simulink library "myLibrary"  (R2023b)
settings: Solver=VariableStepAuto  StartTime=0.0  StopTime=10.0  RelTol=1e-3
undefined symbols (not defined in the file): Cac_n1, ctrl1, Da, delta_slk, Discrete, dtha, ee_sli_rtmsupport, FA, gcbh, Ha, Ini, init_DCline, init_IPC, init_line, init_load, init_SG, init_shunt, init_TH, init_trafo, init_user, init_VSC, initMachineBlocks, Ka, Lf, Llkd_pu, Llkq1_pu, magnitude, NET, P, plots_step, q0, Rac_n1, Radd, Rkd_pu, Rkq1_pu, Rload_add, sim_config, sps_rtmsupport, spsSteamTurbineModel, T_DC_NET, T_global, T_IPC, T_load, T_NET, T_SG, T_shunt, T_STATCOM, T_TH, T_trafo, T_user, T_VSC, Ts, tstep, Udiff_a, V1
libraries: spsSeriesRLCBranchLib x120, eeGeneralControl x83, $bdroot x78, spsCurrentMeasurementLib x53, spsParallelRLCBranchLib x39, spsVoltageMeasurementLib x37, spsControlledVoltageSourceLib x30, simulink x29, spsFirstOrderFilterLib x18, spsMeasurementModel x13, spsThreePhaseVIMeasurementLib x5, dspsigops x4
(part 11 of 16)

== system myLibrary/GFOL/Control/Current Control ==
  Iq* : Inport
  Iq : Inport  Port=2
  Id* : Inport  Port=3
  Id : Inport  Port=4
  uq : Inport  Port=5
  ud : Inport  Port=6
  Constant : Constant  Value=T_VSC.wb
  Id1 : InportShadow  Port=4
  Integrator : Integrator  InitialCondition=initVSC.PI_idiffq
  Integrator1 : Integrator  InitialCondition=initVSC.PI_idiffd
  Iq1 : InportShadow  Port=2
  Ki : Gain  Gain=T_VSC.ki_s
  Ki1 : Gain  Gain=T_VSC.ki_s
  Kp : Gain  Gain=T_VSC.kp_s
  Kp1 : Gain  Gain=T_VSC.kp_s
  Lc : Gain  Gain=T_VSC.Lc
  Product : Product
  Product1 : Product
  Scope : Scope  NumInputPorts=2
  Sum : Sum  Inputs=|+-
  Sum1 : Sum  Inputs=|+-
  Sum2 : Sum  Inputs=+++
  Sum3 : Sum  Inputs=-++
  Sum4 : Sum
  Sum5 : Sum
  V_q_s : Outport  VectorParamsAs1DForOutWhenUnconnected=off
  V_d_s : Outport  Port=2  VectorParamsAs1DForOutWhenUnconnected=off
  wires:
  Sum2/1 -> V_q_s/1
  Sum5/1 -> Sum3/2
  Kp1/1 -> Sum5/2
  Integrator1/1 -> Sum5/1
  Ki1/1 -> Integrator1/1
  Sum1/1 -> Ki1/1, Kp1/1  "Error"
  Kp/1 -> Sum4/2
  Ki/1 -> Integrator/1
  Sum/1 -> Kp/1, Ki/1
  Lc/1 -> Product/2, Product1/1
  Id/1 -> Scope/2, Sum1/2
  Iq/1 -> Sum/2
  Iq*/1 -> Sum/1
  Constant/1 -> Lc/1
  ud/1 -> Sum3/3
  Sum4/1 -> Sum2/1
  uq/1 -> Sum2/3
  Sum3/1 -> V_d_s/1
  Product/1 -> Sum3/1
  Product1/1 -> Sum2/2
  Iq1/1 -> Product/1
  Id1/1 -> Product1/2
  Integrator/1 -> Sum4/1
  Id*/1 -> Scope/1, Sum1/1

== system myLibrary/GFOL/Control/Is ==
  Ias : Inport
  Ibs : Inport  Port=2
  Ics : Inport  Port=3
  Angle : Inport  Port=4
  Demux1 : Demux  Outputs=3
  Matriu T : Subsystem
  Mux : Mux  Inputs=3
  Product : Product  Multiplication=Matrix(*)
  Terminator : Terminator
  I_q_s : Outport  VectorParamsAs1DForOutWhenUnconnected=off
  I_d_s : Outport  Port=2  VectorParamsAs1DForOutWhenUnconnected=off
  wires:
  Product/1 -> Demux1/1
  Matriu T/1(Out1) -> Product/1
  Demux1/1 -> I_q_s/1
  Demux1/2 -> I_d_s/1
  Demux1/3 -> Terminator/1
  Angle/1 -> Matriu T/1(u)
  Mux/1 -> Product/2
  Ias/1 -> Mux/1
  Ibs/1 -> Mux/2
  Ics/1 -> Mux/3

== system myLibrary/GFOL/Control/Is1 ==
  Ias : Inport
  Ibs : Inport  Port=2
  Ics : Inport  Port=3
  Angle : Inport  Port=4
  Demux1 : Demux  Outputs=3
  Matriu T : Subsystem
  Mux : Mux  Inputs=3
  Product : Product  Multiplication=Matrix(*)
  I_q_s : Outport  VectorParamsAs1DForOutWhenUnconnected=off
  I_d_s : Outport  Port=2  VectorParamsAs1DForOutWhenUnconnected=off
  I_0_s : Outport  Port=3  VectorParamsAs1DForOutWhenUnconnected=off
  wires:
  Ics/1 -> Mux/3
  Ibs/1 -> Mux/2
  Ias/1 -> Mux/1
  Mux/1 -> Product/2
  Angle/1 -> Matriu T/1(u)
  Demux1/3 -> I_0_s/1
  Demux1/2 -> I_d_s/1
  Demux1/1 -> I_q_s/1
  Matriu T/1(Out1) -> Product/1
  Product/1 -> Demux1/1

== system myLibrary/GFOL/Control/Is3 ==
  Ias : Inport
  Ibs : Inport  Port=2
  Ics : Inport  Port=3
  Angle : Inport  Port=4
  Demux1 : Demux  Outputs=3
  Matriu T : Subsystem
  Mux : Mux  Inputs=3
  Product : Product  Multiplication=Matrix(*)
  I_q_s : Outport  VectorParamsAs1DForOutWhenUnconnected=off
  I_d_s : Outport  Port=2  VectorParamsAs1DForOutWhenUnconnected=off
  I_0_s : Outport  Port=3  VectorParamsAs1DForOutWhenUnconnected=off
  wires:
  Product/1 -> Demux1/1
  Matriu T/1(Out1) -> Product/1
  Demux1/1 -> I_q_s/1
  Demux1/2 -> I_d_s/1
  Demux1/3 -> I_0_s/1
  Angle/1 -> Matriu T/1(u)
  Mux/1 -> Product/2
  Ias/1 -> Mux/1
  Ibs/1 -> Mux/2
  Ics/1 -> Mux/3

== system myLibrary/GFOL/Control/Is4 ==
  Ias : Inport
  Ibs : Inport  Port=2
  Ics : Inport  Port=3
  Angle : Inport  Port=4
  Demux1 : Demux  Outputs=3
  Matriu T : Subsystem
  Mux : Mux  Inputs=3
  Product : Product  Multiplication=Matrix(*)
  I_q_s : Outport  VectorParamsAs1DForOutWhenUnconnected=off
  I_d_s : Outport  Port=2  VectorParamsAs1DForOutWhenUnconnected=off
  I_0_s : Outport  Port=3  VectorParamsAs1DForOutWhenUnconnected=off
  wires:
  Ics/1 -> Mux/3
  Ibs/1 -> Mux/2
  Ias/1 -> Mux/1
  Mux/1 -> Product/2
  Angle/1 -> Matriu T/1(u)
  Demux1/3 -> I_0_s/1
  Demux1/2 -> I_d_s/1
  Demux1/1 -> I_q_s/1
  Matriu T/1(Out1) -> Product/1
  Product/1 -> Demux1/1

== system myLibrary/GFOL/Control/Is5 ==
  Ias : Inport
  Ibs : Inport  Port=2
  Ics : Inport  Port=3
  Angle : Inport  Port=4
  Demux1 : Demux  Outputs=3
  Matriu T : Subsystem
  Mux : Mux  Inputs=3
  Product : Product  Multiplication=Matrix(*)
  I_q_s : Outport  VectorParamsAs1DForOutWhenUnconnected=off
  I_d_s : Outport  Port=2  VectorParamsAs1DForOutWhenUnconnected=off
  I_0_s : Outport  Port=3  VectorParamsAs1DForOutWhenUnconnected=off
  wires:
  Product/1 -> Demux1/1
  Matriu T/1(Out1) -> Product/1
  Demux1/1 -> I_q_s/1
  Demux1/2 -> I_d_s/1
  Demux1/3 -> I_0_s/1
  Angle/1 -> Matriu T/1(u)
  Mux/1 -> Product/2
  Ias/1 -> Mux/1
  Ibs/1 -> Mux/2
  Ics/1 -> Mux/3

== system myLibrary/GFOL/Control/Is7 ==
  Ias : Inport
  Ibs : Inport  Port=2
  Ics : Inport  Port=3
  Angle : Inport  Port=4
  Demux1 : Demux  Outputs=3
  Matriu T : Subsystem
  Mux : Mux  Inputs=3
  Product : Product  Multiplication=Matrix(*)
  I_q_s : Outport  VectorParamsAs1DForOutWhenUnconnected=off
  I_d_s : Outport  Port=2  VectorParamsAs1DForOutWhenUnconnected=off
  I_0_s : Outport  Port=3  VectorParamsAs1DForOutWhenUnconnected=off
  wires:
  Ics/1 -> Mux/3
  Ibs/1 -> Mux/2
  Ias/1 -> Mux/1
  Mux/1 -> Product/2
  Angle/1 -> Matriu T/1(u)
  Demux1/3 -> I_0_s/1
  Demux1/2 -> I_d_s/1
  Demux1/1 -> I_q_s/1
  Matriu T/1(Out1) -> Product/1
  Product/1 -> Demux1/1

== system myLibrary/GFOL/Control/PLL ==
  note: PLL
  U : Inport
  Ud : Inport  Port=2
  Constant : Constant  Value=0
  Constant1 : Constant
  Demux : Demux  Outputs=3
  Integrator : Integrator  InitialCondition=initVSC.thetaPLL_init
  Integrator1 : Integrator
  Ki : Gain  Gain=T_VSC.ki_pll
  Kp : Gain  Gain=T_VSC.kp_pll
  Scope1 : Scope
  Scope4 : Scope  NumInputPorts=2
  Sum : Sum  Inputs=|+-
  Sum1 : Sum  Inputs=|++
  Sum2 : Sum  Inputs=|++
  Terminator : Terminator
  Tpark : Subsystem
  wb : Gain  Gain=T_VSC.wb
  Angle : Outport
  Vzq : Outport  Port=2
  Vzd : Outport  Port=3
  w : Outport  Port=4
  wires:
  wb/1 -> Integrator/1, w/1
  Sum2/1 -> Scope1/1, wb/1
  Tpark/2(Vd) -> Vzd/1
  Constant1/1 -> Sum2/2
  Sum1/1 -> Sum2/1
  Tpark/3(0) -> Terminator/1
  Integrator/1 -> Angle/1, Tpark/4(u)
  Integrator1/1 -> Sum1/2
  Kp/1 -> Sum1/1
  Ki/1 -> Integrator1/1
  Sum/1 -> Kp/1, Ki/1
  Constant/1 -> Scope4/1, Sum/1
  Demux/1 -> Tpark/1(Va)
  Demux/3 -> Tpark/3(Vc)
  Demux/2 -> Tpark/2(Vb)
  U/1 -> Demux/1
  Tpark/1(Vq) -> Vzq/1
  Ud/1 -> Scope4/2, Sum/2

== system myLibrary/GFOL/Control/Reactive Power Control ==
  Q_ref : Inport
  id : Inport  Port=2
  iq : Inport  Port=3
  Ud : Inport  Port=4
  Uq : Inport  Port=5
  Gain : Gain  Gain=3/2
  Integrator : Integrator  InitialCondition=initVSC.idiffd
  Ki : Gain  Gain=T_VSC.ki_Q
  Kp : Gain  Gain=T_VSC.kp_Q
  Product1 : Product
  Product3 : Product
  Scope : Scope  NumInputPorts=2
  Sum : Sum  Inputs=|+-
  Sum1 : Sum  Inputs=+-
  Sum4 : Sum
  Id_ref : Outport
  wires:
  Sum4/1 -> Id_ref/1
  Sum/1 -> Kp/1, Ki/1
  Ki/1 -> Integrator/1
  Kp/1 -> Sum4/2
  Integrator/1 -> Sum4/1
  Q_ref/1 -> Scope/1, Sum/1
  Sum1/1 -> Gain/1
  Product1/1 -> Sum1/2
  Product3/1 -> Sum1/1
  Ud/1 -> Product1/1
  Uq/1 -> Product3/1
  id/1 -> Product3/2
  iq/1 -> Product1/2
  Gain/1 -> Scope/2, Sum/2

== system myLibrary/GFOL/Control/Rotació ==
  V_q_diff : Inport
  V_d_diff : Inport  Port=2
  V_0_diff : Inport  Port=3
  Angle : Inport  Port=4
  Constant{2,5..7} (4 alike) : Constant  Value=0
  Constant8 : Constant
  Demux : Demux  Outputs=3
  Display : Display
  Gain1 : Gain  Gain=-1
  Matrix Concatenate : Concatenate  NumInputs=3  Mode=Multidimensional array  ConcatenateDimension=2
  Mux{,1..3} (4 alike) : Mux  Inputs=3
  Product : Product  Multiplication=Matrix(*)
  Trigonometric Function : Trigonometry  Operator=cos
  Trigonometric Function1 : Trigonometry
  Trigonometric Function2 : Trigonometry
  Trigonometric Function3 : Trigonometry  Operator=cos
  V_alfa_diff : Outport  VectorParamsAs1DForOutWhenUnconnected=off
  V_beta_diff : Outport  Port=2  VectorParamsAs1DForOutWhenUnconnected=off
  V_0 : Outport  Port=3  VectorParamsAs1DForOutWhenUnconnected=off
  wires:
  Trigonometric Function1/1 -> Gain1/1
  Constant2/1 -> Mux1/3
  Trigonometric Function3/1 -> Mux2/2
  Constant5/1 -> Mux2/3
  Constant6/1 -> Mux3/1
  Constant7/1 -> Mux3/2
  Constant8/1 -> Mux3/3
  Mux2/1 -> Matrix Concatenate/2
  Mux3/1 -> Matrix Concatenate/3
  Mux1/1 -> Matrix Concatenate/1
  Product/1 -> Demux/1
  Demux/1 -> V_alfa_diff/1
  Demux/2 -> V_beta_diff/1
  Demux/3 -> V_0/1
  Mux/1 -> Product/2
  Matrix Concatenate/1 -> Display/1, Product/1
  V_q_diff/1 -> Mux/1
  V_d_diff/1 -> Mux/2
  V_0_diff/1 -> Mux/3
  Trigonometric Function/1 -> Mux1/1
  Gain1/1 -> Mux1/2
  Trigonometric Function2/1 -> Mux2/1
  Angle/1 -> Trigonometric Function/1, Trigonometric Function3/1, Trigonometric Function2/1, Trigonometric Function1/1

== system myLibrary/GFOL_RL/Control/Active Power Control ==
  Pac_ref : Inport
  w : Inport  Port=2
  id : Inport  Port=3
  iq : Inport  Port=4
  Ud : Inport  Port=5
  Uq : Inport  Port=6
  Constant : Constant  Value=T_VSC.wb
  Gain : Gain  Gain=3/2
  Integrator : Integrator  InitialCondition=initVSC.idiffq
  Ki : Gain  Gain=T_VSC.ki_P
  Kp : Gain  Gain=T_VSC.kp_P
  Low-Pass Filter (Discrete or Continuous)4 : eeGeneralControl/Low-Pass Filter (Discrete or Continuous)  K=1  T=T_VSC.tau_droop_f  B=inf  A=-inf  init_option=Specify as parameter  x0=T_VSC.wb  Ts=-1
  Product1 : Product
  Product3 : Product
  Scope : Scope  NumInputPorts=2
  Sum : Sum  Inputs=+-+
  Sum1 : Sum
  Sum2 : Sum  Inputs=|+-
  Sum4 : Sum
  droop : Gain  Gain=T_VSC.k_droop_f/T_VSC.wb
  Iq_ref : Outport
  wires:
  droop/1 -> Sum/3
  w/1 -> Low-Pass Filter (Discrete or Continuous)4/1
  Constant/1 -> Sum2/1
  Sum2/1 -> droop/1
  Low-Pass Filter (Discrete or Continuous)4/1 -> Sum2/2
  Uq/1 -> Product3/1
  iq/1 -> Product3/2
  Ud/1 -> Product1/1
  id/1 -> Product1/2
  Product3/1 -> Sum1/1
  Product1/1 -> Sum1/2
  Sum1/1 -> Gain/1
  Pac_ref/1 -> Scope/1, Sum/1
  Gain/1 -> Scope/2, Sum/2
  Integrator/1 -> Sum4/1
  Kp/1 -> Sum4/2
  Ki/1 -> Integrator/1
  Sum/1 -> Ki/1, Kp/1
  Sum4/1 -> Iq_ref/1

== system myLibrary/GFOL_RL/Control/Clarke Anti-Transformation ==
  V_alfa_diff : Inport
  V_beta_dfff : Inport  Port=2
  V_0_diff : Inport  Port=3
  Constant{,2,5,8} (4 alike) : Constant
  Constant1 : Constant  Value=0
  Constant3 : Constant  Value=-1/2
  Constant4 : Constant  Value=-sqrt(3)/2
  Constant6 : Constant  Value=-1/2
  Constant7 : Constant  Value=sqrt(3)/2
  Demux : Demux  Outputs=3
  Display : Display
  Math Function : Math  Operator=transpose  SignedPower=on
  Matrix Concatenate : Concatenate  NumInputs=3  Mode=Multidimensional array  ConcatenateDimension=2
  Mux{,1..3} (4 alike) : Mux  Inputs=3
  Product : Product  Multiplication=Matrix(*)
  Va_diff : Outport  VectorParamsAs1DForOutWhenUnconnected=off
  Vb_diff : Outport  Port=2  VectorParamsAs1DForOutWhenUnconnected=off
  Vc_diff : Outport  Port=3  VectorParamsAs1DForOutWhenUnconnected=off
  wires:
  Constant/1 -> Mux1/1
  Constant1/1 -> Mux1/2
  Constant2/1 -> Mux1/3
  Constant3/1 -> Mux2/1
  Constant4/1 -> Mux2/2
  Constant5/1 -> Mux2/3
  Constant6/1 -> Mux3/1
  Constant7/1 -> Mux3/2
  Constant8/1 -> Mux3/3
  Matrix Concatenate/1 -> Math Function/1
  Mux2/1 -> Matrix Concatenate/2
  Mux3/1 -> Matrix Concatenate/3
  Mux1/1 -> Matrix Concatenate/1
  Product/1 -> Demux/1
  Demux/1 -> Va_diff/1  "Va"
  Demux/2 -> Vb_diff/1  "Vb"
  Demux/3 -> Vc_diff/1  "Vc"
  Mux/1 -> Product/2
  Math Function/1 -> Display/1, Product/1
  V_alfa_diff/1 -> Mux/1  "Valfa"
  V_beta_dfff/1 -> Mux/2  "Vbeta"
  V_0_diff/1 -> Mux/3  "0"

== system myLibrary/GFOL_RL/Control/Current Control ==
  Iq* : Inport
  Iq : Inport  Port=2
  Id* : Inport  Port=3
  Id : Inport  Port=4
  uq : Inport  Port=5
  ud : Inport  Port=6
  Constant : Constant  Value=T_VSC.wb
  Id1 : InportShadow  Port=4
  Integrator : Integrator  InitialCondition=initVSC.PI_idiffq
  Integrator1 : Integrator  InitialCondition=initVSC.PI_idiffd
  Iq1 : InportShadow  Port=2
  Ki : Gain  Gain=T_VSC.ki_s
  Ki1 : Gain  Gain=T_VSC.ki_s
  Kp : Gain  Gain=T_VSC.kp_s
  Kp1 : Gain  Gain=T_VSC.kp_s
  Lc : Gain  Gain=T_VSC.Lc
  Product : Product
  Product1 : Product
  Scope : Scope  NumInputPorts=2
  Sum : Sum  Inputs=|+-
  Sum1 : Sum  Inputs=|+-
  Sum2 : Sum  Inputs=+++
  Sum3 : Sum  Inputs=-++
  Sum4 : Sum
  Sum5 : Sum
  V_q_s : Outport  VectorParamsAs1DForOutWhenUnconnected=off
  V_d_s : Outport  Port=2  VectorParamsAs1DForOutWhenUnconnected=off
  wires:
  Sum2/1 -> V_q_s/1
  Sum5/1 -> Sum3/2
  Kp1/1 -> Sum5/2
  Integrator1/1 -> Sum5/1
  Ki1/1 -> Integrator1/1
  Sum1/1 -> Ki1/1, Kp1/1  "Error"
  Kp/1 -> Sum4/2
  Ki/1 -> Integrator/1
  Sum/1 -> Kp/1, Ki/1
  Lc/1 -> Product/2, Product1/1
  Id/1 -> Scope/2, Sum1/2
  Iq/1 -> Sum/2
  Iq*/1 -> Sum/1
  Constant/1 -> Lc/1
  ud/1 -> Sum3/3
  Sum4/1 -> Sum2/1
  uq/1 -> Sum2/3
  Sum3/1 -> V_d_s/1
  Product/1 -> Sum3/1
  Product1/1 -> Sum2/2
  Iq1/1 -> Product/1
  Id1/1 -> Product1/2
  Integrator/1 -> Sum4/1
  Id*/1 -> Scope/1, Sum1/1

== system myLibrary/GFOL_RL/Control/Is ==
  Ias : Inport
  Ibs : Inport  Port=2
  Ics : Inport  Port=3
  Angle : Inport  Port=4
  Demux1 : Demux  Outputs=3
  Matriu T : Subsystem
  Mux : Mux  Inputs=3
  Product : Product  Multiplication=Matrix(*)
  Terminator : Terminator
  I_q_s : Outport  VectorParamsAs1DForOutWhenUnconnected=off
  I_d_s : Outport  Port=2  VectorParamsAs1DForOutWhenUnconnected=off
  wires:
  Product/1 -> Demux1/1
  Matriu T/1(Out1) -> Product/1
  Demux1/1 -> I_q_s/1
  Demux1/2 -> I_d_s/1
  Demux1/3 -> Terminator/1
  Angle/1 -> Matriu T/1(u)
  Mux/1 -> Product/2
  Ias/1 -> Mux/1
  Ibs/1 -> Mux/2
  Ics/1 -> Mux/3

== system myLibrary/GFOL_RL/Control/Is1 ==
  Ias : Inport
  Ibs : Inport  Port=2
  Ics : Inport  Port=3
  Angle : Inport  Port=4
  Demux1 : Demux  Outputs=3
  Matriu T : Subsystem
  Mux : Mux  Inputs=3
  Product : Product  Multiplication=Matrix(*)
  I_q_s : Outport  VectorParamsAs1DForOutWhenUnconnected=off
  I_d_s : Outport  Port=2  VectorParamsAs1DForOutWhenUnconnected=off
  I_0_s : Outport  Port=3  VectorParamsAs1DForOutWhenUnconnected=off
  wires:
  Ics/1 -> Mux/3
  Ibs/1 -> Mux/2
  Ias/1 -> Mux/1
  Mux/1 -> Product/2
  Angle/1 -> Matriu T/1(u)
  Demux1/3 -> I_0_s/1
  Demux1/2 -> I_d_s/1
  Demux1/1 -> I_q_s/1
  Matriu T/1(Out1) -> Product/1
  Product/1 -> Demux1/1

== system myLibrary/GFOL_RL/Control/Is3 ==
  Ias : Inport
  Ibs : Inport  Port=2
  Ics : Inport  Port=3
  Angle : Inport  Port=4
  Demux1 : Demux  Outputs=3
  Matriu T : Subsystem
  Mux : Mux  Inputs=3
  Product : Product  Multiplication=Matrix(*)
  I_q_s : Outport  VectorParamsAs1DForOutWhenUnconnected=off
  I_d_s : Outport  Port=2  VectorParamsAs1DForOutWhenUnconnected=off
  I_0_s : Outport  Port=3  VectorParamsAs1DForOutWhenUnconnected=off
  wires:
  Product/1 -> Demux1/1
  Matriu T/1(Out1) -> Product/1
  Demux1/1 -> I_q_s/1
  Demux1/2 -> I_d_s/1
  Demux1/3 -> I_0_s/1
  Angle/1 -> Matriu T/1(u)
  Mux/1 -> Product/2
  Ias/1 -> Mux/1
  Ibs/1 -> Mux/2
  Ics/1 -> Mux/3

== system myLibrary/GFOL_RL/Control/Is4 ==
  Ias : Inport
  Ibs : Inport  Port=2
  Ics : Inport  Port=3
  Angle : Inport  Port=4
  Demux1 : Demux  Outputs=3
  Matriu T : Subsystem
  Mux : Mux  Inputs=3
  Product : Product  Multiplication=Matrix(*)
  I_q_s : Outport  VectorParamsAs1DForOutWhenUnconnected=off
  I_d_s : Outport  Port=2  VectorParamsAs1DForOutWhenUnconnected=off
  I_0_s : Outport  Port=3  VectorParamsAs1DForOutWhenUnconnected=off
  wires:
  Ics/1 -> Mux/3
  Ibs/1 -> Mux/2
  Ias/1 -> Mux/1
  Mux/1 -> Product/2
  Angle/1 -> Matriu T/1(u)
  Demux1/3 -> I_0_s/1
  Demux1/2 -> I_d_s/1
  Demux1/1 -> I_q_s/1
  Matriu T/1(Out1) -> Product/1
  Product/1 -> Demux1/1

== system myLibrary/GFOL_RL/Control/Is5 ==
  Ias : Inport
  Ibs : Inport  Port=2
  Ics : Inport  Port=3
  Angle : Inport  Port=4
  Demux1 : Demux  Outputs=3
  Matriu T : Subsystem
  Mux : Mux  Inputs=3
  Product : Product  Multiplication=Matrix(*)
  I_q_s : Outport  VectorParamsAs1DForOutWhenUnconnected=off
  I_d_s : Outport  Port=2  VectorParamsAs1DForOutWhenUnconnected=off
  I_0_s : Outport  Port=3  VectorParamsAs1DForOutWhenUnconnected=off
  wires:
  Product/1 -> Demux1/1
  Matriu T/1(Out1) -> Product/1
  Demux1/1 -> I_q_s/1
  Demux1/2 -> I_d_s/1
  Demux1/3 -> I_0_s/1
  Angle/1 -> Matriu T/1(u)
  Mux/1 -> Product/2
  Ias/1 -> Mux/1
  Ibs/1 -> Mux/2
  Ics/1 -> Mux/3

== system myLibrary/GFOL_RL/Control/PLL ==
  note: PLL
  U : Inport
  Constant : Constant  Value=0
  Constant1 : Constant
  Demux : Demux  Outputs=3
  Integrator : Integrator  InitialCondition=initVSC.thetaPLL_init
  Integrator1 : Integrator
  Ki : Gain  Gain=T_VSC.ki_pll
  Kp : Gain  Gain=T_VSC.kp_pll
  Scope1 : Scope
  Scope4 : Scope  NumInputPorts=2
  Sum : Sum  Inputs=|+-
  Sum1 : Sum  Inputs=|++
  Sum2 : Sum  Inputs=|++
  Terminator : Terminator
  Tpark : Subsystem
  wb : Gain  Gain=T_VSC.wb
  Angle : Outport
  Vzq : Outport  Port=2
  Vzd : Outport  Port=3
  w : Outport  Port=4
  wires:
  wb/1 -> Integrator/1, w/1
  Sum2/1 -> Scope1/1, wb/1
  Tpark/2(Vd) -> Scope4/2, Sum/2, Vzd/1
  Constant1/1 -> Sum2/2
  Sum1/1 -> Sum2/1
  Tpark/3(0) -> Terminator/1
  Integrator/1 -> Angle/1, Tpark/4(u)
  Integrator1/1 -> Sum1/2
  Kp/1 -> Sum1/1
  Ki/1 -> Integrator1/1
  Sum/1 -> Kp/1, Ki/1
  Constant/1 -> Scope4/1, Sum/1
  Demux/1 -> Tpark/1(Va)
  Demux/3 -> Tpark/3(Vc)
  Demux/2 -> Tpark/2(Vb)
  U/1 -> Demux/1
  Tpark/1(Vq) -> Vzq/1

== system myLibrary/GFOL_RL/Control/Reactive Power Control ==
  Q_ref : Inport
  id : Inport  Port=2
  iq : Inport  Port=3
  Ud : Inport  Port=4
  Uq : Inport  Port=5
  Gain : Gain  Gain=3/2
  Integrator : Integrator  InitialCondition=initVSC.idiffd
  Ki : Gain  Gain=T_VSC.ki_Q
  Kp : Gain  Gain=T_VSC.kp_Q
  Product1 : Product
  Product3 : Product
  Scope : Scope  NumInputPorts=2
  Sum : Sum  Inputs=|+-
  Sum1 : Sum  Inputs=+-
  Sum4 : Sum
  Id_ref : Outport
  wires:
  Sum4/1 -> Id_ref/1
  Sum/1 -> Kp/1, Ki/1
  Ki/1 -> Integrator/1
  Kp/1 -> Sum4/2
  Integrator/1 -> Sum4/1
  Q_ref/1 -> Scope/1, Sum/1
  Sum1/1 -> Gain/1
  Product1/1 -> Sum1/2
  Product3/1 -> Sum1/1
  Ud/1 -> Product1/1
  Uq/1 -> Product3/1
  id/1 -> Product3/2
  iq/1 -> Product1/2
  Gain/1 -> Scope/2, Sum/2

== system myLibrary/GFOL_RL/Control/Rotació ==
  V_q_diff : Inport
  V_d_diff : Inport  Port=2
  V_0_diff : Inport  Port=3
  Angle : Inport  Port=4
  Constant{2,5..7} (4 alike) : Constant  Value=0
  Constant8 : Constant
  Demux : Demux  Outputs=3
  Display : Display
  Gain1 : Gain  Gain=-1
  Matrix Concatenate : Concatenate  NumInputs=3  Mode=Multidimensional array  ConcatenateDimension=2
  Mux{,1..3} (4 alike) : Mux  Inputs=3
  Product : Product  Multiplication=Matrix(*)
  Trigonometric Function : Trigonometry  Operator=cos
  Trigonometric Function1 : Trigonometry
  Trigonometric Function2 : Trigonometry
  Trigonometric Function3 : Trigonometry  Operator=cos
  V_alfa_diff : Outport  VectorParamsAs1DForOutWhenUnconnected=off
  V_beta_diff : Outport  Port=2  VectorParamsAs1DForOutWhenUnconnected=off
  V_0 : Outport  Port=3  VectorParamsAs1DForOutWhenUnconnected=off
  wires:
  Trigonometric Function1/1 -> Gain1/1
  Constant2/1 -> Mux1/3
  Trigonometric Function3/1 -> Mux2/2
  Constant5/1 -> Mux2/3
  Constant6/1 -> Mux3/1
  Constant7/1 -> Mux3/2
  Constant8/1 -> Mux3/3
  Mux2/1 -> Matrix Concatenate/2
  Mux3/1 -> Matrix Concatenate/3
  Mux1/1 -> Matrix Concatenate/1
  Product/1 -> Demux/1
  Demux/1 -> V_alfa_diff/1
  Demux/2 -> V_beta_diff/1
  Demux/3 -> V_0/1
  Mux/1 -> Product/2
  Matrix Concatenate/1 -> Display/1, Product/1
  V_q_diff/1 -> Mux/1
  V_d_diff/1 -> Mux/2
  V_0_diff/1 -> Mux/3
  Trigonometric Function/1 -> Mux1/1
  Gain1/1 -> Mux1/2
  Trigonometric Function2/1 -> Mux2/1
  Angle/1 -> Trigonometric Function/1, Trigonometric Function3/1, Trigonometric Function2/1, Trigonometric Function1/1

== system myLibrary/GFOR/Control/Clarke Anti-Transformation ==
  V_alfa_diff : Inport
  V_beta_dfff : Inport  Port=2
  V_0_diff : Inport  Port=3
  Constant{,2,5,8} (4 alike) : Constant
  Constant1 : Constant  Value=0
  Constant3 : Constant  Value=-1/2
  Constant4 : Constant  Value=-sqrt(3)/2
  Constant6 : Constant  Value=-1/2
  Constant7 : Constant  Value=sqrt(3)/2
  Demux : Demux  Outputs=3
  Display : Display
  Math Function : Math  Operator=transpose  SignedPower=on
  Matrix Concatenate : Concatenate  NumInputs=3  Mode=Multidimensional array  ConcatenateDimension=2
  Mux{,1..3} (4 alike) : Mux  Inputs=3
  Product : Product  Multiplication=Matrix(*)
  Va_diff : Outport  VectorParamsAs1DForOutWhenUnconnected=off
  Vb_diff : Outport  Port=2  VectorParamsAs1DForOutWhenUnconnected=off
  Vc_diff : Outport  Port=3  VectorParamsAs1DForOutWhenUnconnected=off
  wires:
  V_0_diff/1 -> Mux/3  "0"
  V_beta_dfff/1 -> Mux/2  "Vbeta"
  V_alfa_diff/1 -> Mux/1  "Valfa"
  Math Function/1 -> Product/1, Display/1
  Mux/1 -> Product/2
  Demux/3 -> Vc_diff/1  "Vc"
  Demux/2 -> Vb_diff/1  "Vb"
  Demux/1 -> Va_diff/1  "Va"
  Product/1 -> Demux/1
  Mux1/1 -> Matrix Concatenate/1
  Mux3/1 -> Matrix Concatenate/3
  Mux2/1 -> Matrix Concatenate/2
  Matrix Concatenate/1 -> Math Function/1
  Constant8/1 -> Mux3/3
  Constant7/1 -> Mux3/2
  Constant6/1 -> Mux3/1
  Constant5/1 -> Mux2/3
  Constant4/1 -> Mux2/2
  Constant3/1 -> Mux2/1
  Constant2/1 -> Mux1/3
  Constant1/1 -> Mux1/2
  Constant/1 -> Mux1/1

== system myLibrary/GFOR/Control/Current Control ==
  Iq* : Inport
  Iq : Inport  Port=2
  Id* : Inport  Port=3
  Id : Inport  Port=4
  uq : Inport  Port=5
  ud : Inport  Port=6
  Constant : Constant  Value=T_VSC.wb
  Id1 : InportShadow  Port=4
  Integrator : Integrator  InitialCondition=initVSC.PI_idiffq
  Integrator1 : Integrator  InitialCondition=initVSC.PI_idiffd
  Iq1 : InportShadow  Port=2
  Ki : Gain  Gain=T_VSC.ki_s
  Ki1 : Gain  Gain=T_VSC.ki_s
  Kp : Gain  Gain=T_VSC.kp_s
  Kp1 : Gain  Gain=T_VSC.kp_s
  Lc : Gain  Gain=T_VSC.Lc
  Product : Product
  Product1 : Product
  Sum : Sum  Inputs=|+-
  Sum1 : Sum  Inputs=|+-
  Sum2 : Sum  Inputs=+++
  Sum3 : Sum  Inputs=-++
  Sum4 : Sum
  Sum5 : Sum
  V_q_s : Outport  VectorParamsAs1DForOutWhenUnconnected=off
  V_d_s : Outport  Port=2  VectorParamsAs1DForOutWhenUnconnected=off
  wires:
  Id*/1 -> Sum1/1
  Integrator/1 -> Sum4/1
  Id1/1 -> Product1/2
  Iq1/1 -> Product/1
  Product1/1 -> Sum2/2
  Product/1 -> Sum3/1
  Sum3/1 -> V_d_s/1
  uq/1 -> Sum2/3
  Sum4/1 -> Sum2/1
  ud/1 -> Sum3/3
  Constant/1 -> Lc/1
  Iq*/1 -> Sum/1
  Iq/1 -> Sum/2
  Id/1 -> Sum1/2
  Lc/1 -> Product1/1, Product/2
  Sum/1 -> Ki/1, Kp/1
  Ki/1 -> Integrator/1
  Kp/1 -> Sum4/2
  Sum1/1 -> Kp1/1, Ki1/1  "Error"
  Ki1/1 -> Integrator1/1
  Integrator1/1 -> Sum5/1
  Kp1/1 -> Sum5/2
  Sum5/1 -> Sum3/2
  Sum2/1 -> V_q_s/1

== system myLibrary/GFOR/Control/Is ==
  Ias : Inport
  Ibs : Inport  Port=2
  Ics : Inport  Port=3
  Angle : Inport  Port=4
  Demux1 : Demux  Outputs=3
  Matriu T : Subsystem
  Mux : Mux  Inputs=3
  Product : Product  Multiplication=Matrix(*)
  Terminator : Terminator
  I_q_s : Outport  VectorParamsAs1DForOutWhenUnconnected=off
  I_d_s : Outport  Port=2  VectorParamsAs1DForOutWhenUnconnected=off
  wires:
  Ics/1 -> Mux/3
  Ibs/1 -> Mux/2
  Ias/1 -> Mux/1
  Mux/1 -> Product/2
  Angle/1 -> Matriu T/1(u)
  Demux1/3 -> Terminator/1
  Demux1/2 -> I_d_s/1
  Demux1/1 -> I_q_s/1
  Matriu T/1(Out1) -> Product/1
  Product/1 -> Demux1/1

== system myLibrary/GFOR/Control/Is2 ==
  Ias : Inport
  Ibs : Inport  Port=2
  Ics : Inport  Port=3
  Angle : Inport  Port=4
  Demux1 : Demux  Outputs=3
  Matriu T : Subsystem
  Mux : Mux  Inputs=3
  Product : Product  Multiplication=Matrix(*)
  I_q_s : Outport  VectorParamsAs1DForOutWhenUnconnected=off
  I_d_s : Outport  Port=2  VectorParamsAs1DForOutWhenUnconnected=off
  I_0_s : Outport  Port=3  VectorParamsAs1DForOutWhenUnconnected=off
  wires:
  Ics/1 -> Mux/3
  Ibs/1 -> Mux/2
  Ias/1 -> Mux/1
  Mux/1 -> Product/2
  Angle/1 -> Matriu T/1(u)
  Demux1/3 -> I_0_s/1
  Demux1/2 -> I_d_s/1
  Demux1/1 -> I_q_s/1
  Matriu T/1(Out1) -> Product/1
  Product/1 -> Demux1/1

== system myLibrary/GFOR/Control/PLL ==
  note: PLL
  Pref : Inport
  iq : Inport  Port=2
  uq : Inport  Port=3
  id : Inport  Port=4
  ud : Inport  Port=5
  Constant4 : Constant
  Gain5 : Gain  Gain=3/2
  Integrator2 : Integrator  InitialCondition=initVSC.thetaPLL_init
  Low-Pass Filter (Discrete or Continuous)2 : eeGeneralControl/Low-Pass Filter (Discrete or Continuous)  K=1  T=T_VSC.tau_droop_f  B=inf  A=-inf  init_option=Specify as parameter  x0=initVSC.Pref  Ts=0
  Product3 : Product
  Product5 : Product
  Scope4 : Scope  NumInputPorts=2
  Sum18 : Sum  Inputs=++|
  Sum3 : Sum
  Sum35 : Sum  Inputs=|+-
  kdroop : Gain  Gain=T_VSC.k_droop_f
  wb : Gain  Gain=T_VSC.wb
  Angle : Outport
  tag scope: w_GFOR1=global
  wires:
  Product5/1 -> Sum3/2
  Low-Pass Filter (Discrete or Continuous)2/1 -> Scope4/1, Sum35/2
  Product3/1 -> Sum3/1
  Sum35/1 -> kdroop/1
  Sum18/1 -> wb/1
  Integrator2/1 -> Angle/1
  Sum3/1 -> Gain5/1  "V_0_s"
  Constant4/1 -> Sum18/1  "w0_pu"
  kdroop/1 -> Sum18/2
  Gain5/1 -> Low-Pass Filter (Discrete or Continuous)2/1
  iq/1 -> Product3/1
  uq/1 -> Product3/2
  id/1 -> Product5/1
  ud/1 -> Product5/2
  Pref/1 -> Sum35/1, Scope4/2
  wb/1 -> [w_GFOR1], Integrator2/1

== system myLibrary/GFOR/Control/Rotació ==
  V_q_diff : Inport
  V_d_diff : Inport  Port=2
  V_0_diff : Inport  Port=3
  Angle : Inport  Port=4
  Constant{2,5..7} (4 alike) : Constant  Value=0
  Constant8 : Constant
  Demux : Demux  Outputs=3
  Display : Display
  Gain1 : Gain  Gain=-1
  Matrix Concatenate : Concatenate  NumInputs=3  Mode=Multidimensional array  ConcatenateDimension=2
  Mux{,1..3} (4 alike) : Mux  Inputs=3
  Product : Product  Multiplication=Matrix(*)
  Trigonometric Function : Trigonometry  Operator=cos
  Trigonometric Function1 : Trigonometry
  Trigonometric Function2 : Trigonometry
  Trigonometric Function3 : Trigonometry  Operator=cos
  V_alfa_diff : Outport  VectorParamsAs1DForOutWhenUnconnected=off
  V_beta_diff : Outport  Port=2  VectorParamsAs1DForOutWhenUnconnected=off
  V_0 : Outport  Port=3  VectorParamsAs1DForOutWhenUnconnected=off
  wires:
  Angle/1 -> Trigonometric Function1/1, Trigonometric Function2/1, Trigonometric Function3/1, Trigonometric Function/1
  Trigonometric Function2/1 -> Mux2/1
  Gain1/1 -> Mux1/2
  Trigonometric Function/1 -> Mux1/1
  V_0_diff/1 -> Mux/3
  V_d_diff/1 -> Mux/2
  V_q_diff/1 -> Mux/1
  Matrix Concatenate/1 -> Product/1, Display/1
  Mux/1 -> Product/2
  Demux/3 -> V_0/1
  Demux/2 -> V_beta_diff/1
  Demux/1 -> V_alfa_diff/1
  Product/1 -> Demux/1
  Mux1/1 -> Matrix Concatenate/1
  Mux3/1 -> Matrix Concatenate/3
  Mux2/1 -> Matrix Concatenate/2
  Constant8/1 -> Mux3/3
  Constant7/1 -> Mux3/2
  Constant6/1 -> Mux3/1
  Constant5/1 -> Mux2/3
  Trigonometric Function3/1 -> Mux2/2
  Constant2/1 -> Mux1/3
  Trigonometric Function1/1 -> Gain1/1

== system myLibrary/GFOR/Control/Voltage control ==
  vq_ref : Inport
  vd_ref : Inport  Port=2
  vq : Inport  Port=3
  vd : Inport  Port=4
  igq : Inport  Port=5
  igd : Inport  Port=6
  Cac : Gain  Gain=T_VSC.Cac
  Constant : Constant  Value=T_VSC.wb
  Feed-Forward filter igq : eeGeneralControl/Low-Pass Filter (Discrete or Continuous)  K=1  T=T_VSC.tau_ig  B=inf  A=-inf  init_option=Specify as parameter  x0=initVSC.igq  Ts=0
  Feed-Forward filter igq1 : eeGeneralControl/Low-Pass Filter (Discrete or Continuous)  K=1  T=T_VSC.tau_ig  B=inf  A=-inf  init_option=Specify as parameter  x0=initVSC.igd  Ts=0
  Integrator1 : Integrator  InitialCondition=initVSC.PI_vacq
  Integrator2 : Integrator  InitialCondition=initVSC.PI_vacd
  Product3 : Product  RndMeth=Zero
  Product4 : Product  RndMeth=Zero
  Scope : Scope  NumInputPorts=2
  Sum1 : Sum  Inputs=|+-
  Sum10 : Sum  Inputs=|++
  Sum2 : Sum  Inputs=+++
  Sum3 : Sum  Inputs=-+|
  Sum5 : Sum  Inputs=-++
  Sum8 : Sum  Inputs=|++
  ki : Gain  Gain=T_VSC.ki_vac
  ki2 : Gain  Gain=T_VSC.ki_vac
  kp : Gain  Gain=T_VSC.kp_vac
  kp2 : Gain  Gain=T_VSC.kp_vac
  vd1 : InportShadow  Port=4
  vq1 : InportShadow  Port=3
  iqref : Outport  VectorParamsAs1DForOutWhenUnconnected=off
  idref : Outport  Port=2  VectorParamsAs1DForOutWhenUnconnected=off
  wires:
  vd1/1 -> Product4/2
  vq1/1 -> Product3/1
  Sum8/1 -> Sum2/2
  vd/1 -> Sum3/1
  vq/1 -> Sum1/2
  ki2/1 -> Integrator2/1
  kp2/1 -> Sum10/1
  ki/1 -> Integrator1/1
  vd_ref/1 -> Sum3/2
  Sum5/1 -> idref/1
  vq_ref/1 -> Sum1/1
  Integrator1/1 -> Scope/1, Sum8/2
  Sum10/1 -> Sum5/2
  kp/1 -> Sum8/1
  Integrator2/1 -> Sum10/2, Scope/2
  Sum2/1 -> iqref/1
  Constant/1 -> Cac/1
  Cac/1 -> Product4/1, Product3/2
  Sum1/1 -> ki/1, kp/1
  Sum3/1 -> ki2/1, kp2/1
  Product3/1 -> Sum5/1
  Product4/1 -> Sum2/3
  Feed-Forward filter igq/1 -> Sum2/1
  Feed-Forward filter igq1/1 -> Sum5/3
  igd/1 -> Feed-Forward filter igq1/1
  igq/1 -> Feed-Forward filter igq/1

== system myLibrary/SG/Exciter/Exciter AC4A ==
  vref : Inport
  Vt : Inport  Port=2
  Vs : Inport  Port=3
  IC1 : InitialCondition  Value=0
  Lag-lead network Transient gain reduction : TransferFcn  Numerator=[T_SG.exc.TC 1]  Denominator=[T_SG.exc.TB 1]
  Sum2 : Sum  Inputs=+-+
  Transfer Fcn3 : TransferFcn  Numerator=[T_SG.exc.KA]  Denominator=[T_SG.exc.TA 1]
  Voltage transducer : spsFirstOrderFilterLib/First-Order Filter  FilterType=Lowpass  Tc=T_SG.exc.TR  Ts=sim_config.Ts  Initialize=on  Vac_Init=[0, 0, T_SG.fb]  Vdc_Init=initSG.Vref  PlotResponse=off  FreqRange="[0,  200,  1]"
  Vfn_pu : Outport
  wires:
  Vs/1 -> Sum2/3  "V"
  Voltage transducer/1 -> Sum2/2  "Vc"
  Vt/1 -> Voltage transducer/1  "V"
  Sum2/1 -> IC1/1  "VI"
  Lag-lead network Transient gain reduction/1 -> Transfer Fcn3/1  "VR"
  vref/1 -> Sum2/1
  Transfer Fcn3/1 -> Vfn_pu/1  "Vfn_pu"
  IC1/1 -> Lag-lead network Transient gain reduction/1

== system myLibrary/SG/Exciter/Exciter AC8C ==
  vref : Inport
  Vs : Inport  Port=2
  Vt : Inport  Port=3
  Ifd_pu : Inport  Port=4
  AC ROTATING MACHINE : Subsystem
  Divide : Product  Inputs=*/
  Gain : Gain  Gain=T_SG.exc.KP
  Gain1 : Gain  Gain=-0.577*T_SG.exc.KC  OutDataTypeStr=double
  Lag-lead network Transient gain reduction2 : TransferFcn  Numerator=[(T_SG.exc.KPR*T_SG.exc.TDR+T_SG.exc.KDR) (T_SG.exc.KPR+T_SG.exc.KIR*T_SG.exc.TDR) (T_SG.exc.KIR)]  Denominator=[T_SG.exc.TDR 1 0]
  Product : Product  OutDataTypeStr=Inherit: Same as first input
  Product1 : Product
  Sum : Sum  Inputs=+-+  InputSameDT=on  SaturateOnIntegerOverflow=on  OutDataTypeStr=Inherit: Same as first input
  Transfer Fcn3 : TransferFcn  Numerator=[T_SG.exc.KA]  Denominator=[T_SG.exc.TA 1]
  Voltage transducer : spsFirstOrderFilterLib/First-Order Filter  FilterType=Lowpass  Tc=T_SG.exc.TR  Ts=sim_config.Ts  Initialize=on  Vac_Init=[0, 0, T_SG.fb]  Vdc_Init=initSG.Vref  PlotResponse=off  FreqRange="[0,  200,  1]"
  Vt1 : InportShadow  Port=3
  Vfn_pu : Outport
  wires:
  Product1/1 -> Product/2  "V_B"
  Sum/1 -> Lag-lead network Transient gain reduction2/1  "VR"
  Vt/1 -> Voltage transducer/1  "V"
  Vt1/1 -> Gain/1  "V"
  Vs/1 -> Sum/3
  Gain/1 -> Divide/2, Product1/2  "V_E"
  Gain1/1 -> Product1/1  "F_EX"
  vref/1 -> Sum/1
  Voltage transducer/1 -> Sum/2  "Vc"
  Lag-lead network Transient gain reduction2/1 -> Transfer Fcn3/1  "V_M"
  Product/1 -> AC ROTATING MACHINE/1(EFE)
  Ifd_pu/1 -> AC ROTATING MACHINE/2(IFD)
  AC ROTATING MACHINE/2(VFE) -> Divide/1
  AC ROTATING MACHINE/1(EFD) -> Vfn_pu/1
  Divide/1 -> Gain1/1  "F_EX"
  Transfer Fcn3/1 -> Product/1  "V_A"

== system myLibrary/SG/Exciter/Exciter ST1 ==
  vref : Inport
  Vt : Inport  Port=2
  Vs : Inport  Port=3
  IC1 : InitialCondition  Value=0
  Lag-lead network Transient gain reduction : TransferFcn  Numerator=[T_SG.exc.TC 1]  Denominator=[T_SG.exc.TB 1]
  Sum2 : Sum  Inputs=+-+
  Transfer Fcn3 : TransferFcn  Numerator=[T_SG.exc.KA]  Denominator=[T_SG.exc.TA 1]
  Voltage transducer : spsFirstOrderFilterLib/First-Order Filter  FilterType=Lowpass  Tc=T_SG.exc.TR  Ts=sim_config.Ts  Initialize=on  Vac_Init=[0, 0, T_SG.fb]  Vdc_Init=initSG.Vref  PlotResponse=off  FreqRange="[0,  200,  1]"
  Vfn_pu : Outport
  wires:
  Vs/1 -> Sum2/3  "V"
  Voltage transducer/1 -> Sum2/2  "Vc"
  Vt/1 -> Voltage transducer/1  "V"
  Sum2/1 -> IC1/1  "VI"
  Lag-lead network Transient gain reduction/1 -> Transfer Fcn3/1  "VR"
  vref/1 -> Sum2/1
  Transfer Fcn3/1 -> Vfn_pu/1  "Vfn_pu"
  IC1/1 -> Lag-lead network Transient gain reduction/1

== system myLibrary/SG/Exciter/Exciter ST4B ==
  note: Excitation
      | Control
      | Elements
  V_REF : Inport  SampleTime=Ts
  V_S : Inport  Port=2  SampleTime=Ts
  V_T : Inport  Port=3  SampleTime=Ts
  Ifd_pu : Inport  Port=4  SampleTime=Ts
  Fex : Subsystem  mask{K_C=K_C}
      mask prompts: K_C "Rectifier regulation factor, K_C (pu):"
  PI_M : Subsystem
  PI_R : Subsystem
  Product : Product  OutDataTypeStr=Inherit: Same as first input
  Product1 : Product
  Subsystem1 : Subsystem
      mask Display: disp('V_E=|K_P*V_T+j(K_I+K_P*X_L)*I_T|')
  Sum : Sum  Inputs=+-+  InputSameDT=on  SaturateOnIntegerOverflow=on  OutDataTypeStr=Inherit: Same as first input
  Transfer Fcn3 : TransferFcn  Denominator=[T_SG.exc.TA 1]
  V_T1 : InportShadow  Port=3  SampleTime=Ts
  Voltage transducer : spsFirstOrderFilterLib/First-Order Filter  FilterType=Lowpass  Tc=T_SG.exc.TR  Ts=sim_config.Ts  Initialize=on  Vac_Init=[0, 0, T_SG.fb]  Vdc_Init=initSG.Vref  PlotResponse=off  FreqRange="[0,  200,  1]"
  Efd_pu : Outport  VectorParamsAs1DForOutWhenUnconnected=off
  wires:
  V_REF/1 -> Sum/1
  V_T/1 -> Voltage transducer/1
  Sum/1 -> PI_R/1(u)
  Transfer Fcn3/1 -> Product/1  "V_A"
  Product/1 -> Efd_pu/1
  Fex/1(F_EX) -> Product1/1  "F_EX"
  V_T1/1 -> Subsystem1/1(V_T)
  Ifd_pu/1 -> Fex/2(Ifd)
  Subsystem1/1(y) -> Product1/2, Fex/1(V_E)  "V_E"
  Product1/1 -> Product/2  "V_B"
  V_S/1 -> Sum/3
  Voltage transducer/1 -> Sum/2  "Vc"
  PI_R/1(y) -> PI_M/1(u)  "V_R"
  PI_M/1(y) -> Transfer Fcn3/1  "V_M"

== system myLibrary/SG/Exciter/Exciter ST4C ==
  vref : Inport
  Vs : Inport  Port=2
  Vt : Inport  Port=3
  Ifd_pu : Inport  Port=4
  Fex : $bdroot/SG/Exciter/Exciter ST4B/Fex  K_C=T_SG.exc.KC
  Gain : Gain  Gain=T_SG.exc.KP
  Lag-lead network Transient gain reduction1 : TransferFcn  Numerator=[T_SG.exc.KPR T_SG.exc.KIR]  Denominator=[1 0]
  Lag-lead network Transient gain reduction2 : TransferFcn  Numerator=[T_SG.exc.KPM T_SG.exc.KIM]  Denominator=[1 0]
  Lag-lead network Transient gain reduction3 : TransferFcn  Numerator=[T_SG.exc.KG]  Denominator=[T_SG.exc.TG 1]
  Product : Product  OutDataTypeStr=Inherit: Same as first input
  Product1 : Product
  Sum : Sum  Inputs=+-+  InputSameDT=on  SaturateOnIntegerOverflow=on  OutDataTypeStr=Inherit: Same as first input
  Sum1 : Sum  Inputs=-+|
  Transfer Fcn3 : TransferFcn  Denominator=[T_SG.exc.TA 1]
  Voltage transducer : spsFirstOrderFilterLib/First-Order Filter  FilterType=Lowpass  Tc=T_SG.exc.TR  Ts=sim_config.Ts  Initialize=on  Vac_Init=[0, 0, T_SG.fb]  Vdc_Init=initSG.Vref  PlotResponse=off  FreqRange="[0,  200,  1]"
  Vt1 : InportShadow  Port=3
  Vfn_pu : Outport
  wires:
  Lag-lead network Transient gain reduction2/1 -> Transfer Fcn3/1  "V_M"
  Voltage transducer/1 -> Sum/2  "Vc"
  Product/1 -> Lag-lead network Transient gain reduction3/1, Vfn_pu/1
  vref/1 -> Sum/1
  Transfer Fcn3/1 -> Product/1  "V_A"
  Ifd_pu/1 -> Fex/2
  Fex/1 -> Product1/1  "F_EX"
  Gain/1 -> Product1/2, Fex/1  "V_E"
  Sum/1 -> Lag-lead network Transient gain reduction1/1
  Vs/1 -> Sum/3
  Vt1/1 -> Gain/1  "V"
  Vt/1 -> Voltage transducer/1  "V"
  Lag-lead network Transient gain reduction1/1 -> Sum1/2  "VR"
  Sum1/1 -> Lag-lead network Transient gain reduction2/1
  Lag-lead network Transient gain reduction3/1 -> Sum1/1  "VR"
  Product1/1 -> Product/2  "V_B"

== system myLibrary/SG/Exciter/PSS 2A ==
  Vsi1 : Inport
  Vsi2 : Inport  Port=2
  DW{,1..5,7..8} (8 alike) : Scope
  Gain : Gain  Gain=ks3
  Gain1 : Gain  Gain=ks1
  LTI System1 : cstblocks/LTI System  sys=(tf([T8 1],1)/(tf([T9 1],1)^M))^N  IC=[]  PadeOrder=0
  Ramp-Tracking Filter : eeSmPSS2C/SM PSS2C/Ramp-Tracking Filter  Commented=on  T1=T_8  T2=T_9  M=M  N=N  Ts=Ts
  Sum : Sum  Inputs=|++
  Sum1 : Sum  Inputs=|+-
  Transfer Fcn : TransferFcn  Numerator="[Tw1  0]"  Denominator="[Tw1  1]"
  Transfer Fcn1 : TransferFcn  Numerator="[Tw2  0]"  Denominator=[Tw2 1]
  Transfer Fcn2 : TransferFcn  Numerator=[Tw3 0]  Denominator=[Tw3 1]
  Transfer Fcn3 : TransferFcn  Denominator=[T6 1]
  Transfer Fcn8 : TransferFcn  Numerator=[ks2]  Denominator="[T7  1]"
  t1,t2 : TransferFcn  Numerator=[T1 1]  Denominator=[T2 1]
  t3,t4 : TransferFcn  Numerator=[T3 1]  Denominator=[T4 1]
  Vst : Outport
  wires:
  Transfer Fcn3/1 -> DW8/1, Sum/1
  Transfer Fcn/1 -> Transfer Fcn1/1
  Vsi2/1 -> Transfer Fcn2/1
  Gain/1 -> Sum/2
  Transfer Fcn8/1 -> Sum1/2, Gain/1, DW1/1
  Transfer Fcn1/1 -> Transfer Fcn3/1
  Transfer Fcn2/1 -> Transfer Fcn8/1
  t3,t4/1 -> DW5/1, Vst/1
  Gain1/1 -> t1,t2/1, DW3/1
  t1,t2/1 -> t3,t4/1, DW4/1
  Sum/1 -> DW/1, LTI System1/1
  LTI System1/1 -> DW2/1, Sum1/1
  Vsi1/1 -> DW7/1, Transfer Fcn/1
  Sum1/1 -> Gain1/1

== system myLibrary/SG/Exciter/Terminal voltage magnitude ==
  Vq : Inport
  Vd : Inport  Port=2
  Add10 : Sum
  Product : Product
  Product1 : Product
  Square Root : Sqrt
  Vt : Outport
  wires:
  Product/1 -> Add10/1
  Vd/1 -> Product1/2, Product1/1
  Product1/1 -> Add10/2
  Add10/1 -> Square Root/1
  Vq/1 -> Product/1, Product/2
  Square Root/1 -> Vt/1  "V"

== system myLibrary/SG/Governor-Turbine/IEEEG1 ==
  speed_pu : Inport  SampleTime=Ts
  Pref : Inport  Port=2  SampleTime=Ts
  Add1 : Sum
  Constant : Constant  Value=pu_speed_reference
  Gain : Gain  Gain=K
  Gain10 : Gain  Gain=1/T_3
  Gain2 : Gain  Gain=K_2
  Gain3 : Gain  Gain=K_4
  Gain4 : Gain  Gain=K_6
  Gain5 : Gain  Gain=K_8
  Gain6 : Gain  Gain=K_1
  Gain7 : Gain  Gain=K_3
  Gain8 : Gain  Gain=K_5
  Gain9 : Gain  Gain=K_7
  Integrator : Integrator  InitialCondition=pu_torque0
  Lead-Lag : eeGeneralControl/Lead-Lag (Discrete or Continuous)  T1=T_2  T2=T_1  B=inf  A=-inf  init_option=Inherited from block input  x0=0  Ts=Ts
  Low-Pass Filter : eeGeneralControl/Low-Pass Filter (Discrete or Continuous)  K=1  T=T_4  B=inf  A=-inf  init_option=Inherited from block input  x0=0  Ts=Ts
  Low-Pass Filter1 : eeGeneralControl/Low-Pass Filter (Discrete or Continuous)  K=1  T=T_5  B=inf  A=-inf  init_option=Inherited from block input  x0=0  Ts=Ts
  Low-Pass Filter2 : eeGeneralControl/Low-Pass Filter (Discrete or Continuous)  K=1  T=T_6  B=inf  A=-inf  init_option=Inherited from block input  x0=0  Ts=Ts
  Low-Pass Filter3 : eeGeneralControl/Low-Pass Filter (Discrete or Continuous)  K=1  T=T_7  B=inf  A=-inf  init_option=Inherited from block input  x0=0  Ts=Ts
  Sum1 : Sum  Inputs=++-
  Sum2 : Sum  Inputs=|-+  OutDataTypeStr=Inherit: Same as first input
  Sum3 : Sum  Inputs=++|
  Sum4 : Sum  Inputs=++|
  Sum5 : Sum  Inputs=++|
  Sum6 : Sum  Inputs=|++
  Sum7 : Sum  Inputs=|++
  Sum8 : Sum  Inputs=|++
  Pm(HP) : Outport  VectorParamsAs1DForOutWhenUnconnected=off
  Pm(LP) : Outport  Port=2  VectorParamsAs1DForOutWhenUnconnected=off
  Pm : Outport  Port=3  VectorParamsAs1DForOutWhenUnconnected=off
  wires:
  Add1/1 -> Pm/1  "Pm"
  Gain10/1 -> Integrator/1
  Sum1/1 -> Gain10/1
  Constant/1 -> Sum2/2
  speed_pu/1 -> Sum2/1
  Sum5/1 -> Pm(LP)/1, Add1/2
  Sum8/1 -> Pm(HP)/1, Add1/1
  Sum7/1 -> Sum8/1
  Gain9/1 -> Sum8/2
  Sum6/1 -> Sum7/1
  Gain8/1 -> Sum7/2
  Gain5/1 -> Sum5/1
  Sum4/1 -> Sum5/2
  Sum3/1 -> Sum4/2
  Gain4/1 -> Sum4/1
  Gain2/1 -> Sum3/2
  Gain3/1 -> Sum3/1
  Gain7/1 -> Sum6/2
  Gain6/1 -> Sum6/1
  Low-Pass Filter3/1 -> Gain9/1, Gain5/1
  Low-Pass Filter1/1 -> Low-Pass Filter2/1, Gain3/1, Gain7/1
  Low-Pass Filter2/1 -> Low-Pass Filter3/1, Gain4/1, Gain8/1
  Low-Pass Filter/1 -> Gain2/1, Low-Pass Filter1/1, Gain6/1
  Pref/1 -> Sum1/1
  Integrator/1 -> Low-Pass Filter/1, Sum1/3
  Lead-Lag/1 -> Sum1/2
  Gain/1 -> Lead-Lag/1
  Sum2/1 -> Gain/1

== system myLibrary/SG/Governor-Turbine/Steam Turbine and Governor ==
  wref : Inport
  Pref : Inport  Port=2
  wm : Inport  Port=3
  d_theta : Inport  Port=4
  Model : Subsystem  AncestorBlock=spsSteamTurbineModel/Discrete  DialogController=POWERSYS.PowerSysDialog
      settings: LibrarySourceBlock=spsSteamTurbineModel/Discrete
  dw_5-2 : Outport  VectorParamsAs1DForOutWhenUnconnected=off
  Tr5-2 : Outport  Port=2  VectorParamsAs1DForOutWhenUnconnected=off
  gate : Outport  Port=3  VectorParamsAs1DForOutWhenUnconnected=off
  Pm : Outport  Port=4  VectorParamsAs1DForOutWhenUnconnected=off
  wires:
  wm/1 -> Model/4(wm)
  Model/4(gate) -> gate/1
  Model/3(dw_5-2) -> dw_5-2/1
  d_theta/1 -> Model/3(d_theta)
  Model/2(Tr5-2) -> Tr5-2/1
  Model/1(Pm) -> Pm/1
  wref/1 -> Model/2(wref)
  Pref/1 -> Model/1(Pref)

== system myLibrary/SG_step/Exciter/Exciter AC4A ==
  vref : Inport
  Vt : Inport  Port=2
  Vs : Inport  Port=3
  IC1 : InitialCondition  Value=0
  Lag-lead network Transient gain reduction : TransferFcn  Numerator=[T_SG.exc.TC 1]  Denominator=[T_SG.exc.TB 1]
  Sum2 : Sum  Inputs=+-+
  Transfer Fcn3 : TransferFcn  Numerator=[T_SG.exc.KA]  Denominator=[T_SG.exc.TA 1]
  Voltage transducer : spsFirstOrderFilterLib/First-Order Filter  FilterType=Lowpass  Tc=T_SG.exc.TR  Ts=sim_config.Ts  Initialize=on  Vac_Init=[0, 0, T_SG.fb]  Vdc_Init=initSG.Vref  PlotResponse=off  FreqRange="[0,  200,  1]"
  Vfn_pu : Outport
  wires:
  Vs/1 -> Sum2/3  "V"
  Voltage transducer/1 -> Sum2/2  "Vc"
  Vt/1 -> Voltage transducer/1  "V"
  Sum2/1 -> IC1/1  "VI"
  Lag-lead network Transient gain reduction/1 -> Transfer Fcn3/1  "VR"
  vref/1 -> Sum2/1
  Transfer Fcn3/1 -> Vfn_pu/1  "Vfn_pu"
  IC1/1 -> Lag-lead network Transient gain reduction/1

== system myLibrary/SG_step/Exciter/Exciter ST1 ==
  vref : Inport
  Vt : Inport  Port=2
  Vs : Inport  Port=3
  IC1 : InitialCondition  Value=0
  Lag-lead network Transient gain reduction : TransferFcn  Numerator=[T_SG.exc.TC 1]  Denominator=[T_SG.exc.TB 1]
  Sum2 : Sum  Inputs=+-+
  Transfer Fcn3 : TransferFcn  Numerator=[T_SG.exc.KA]  Denominator=[T_SG.exc.TA 1]
  Voltage transducer : spsFirstOrderFilterLib/First-Order Filter  FilterType=Lowpass  Tc=T_SG.exc.TR  Ts=sim_config.Ts  Initialize=on  Vac_Init=[0, 0, T_SG.fb]  Vdc_Init=initSG.Vref  PlotResponse=off  FreqRange="[0,  200,  1]"
  Vfn_pu : Outport
  wires:
  Vs/1 -> Sum2/3  "V"
  Voltage transducer/1 -> Sum2/2  "Vc"
  Vt/1 -> Voltage transducer/1  "V"
  Sum2/1 -> IC1/1  "VI"
  Lag-lead network Transient gain reduction/1 -> Transfer Fcn3/1  "VR"
  vref/1 -> Sum2/1
  Transfer Fcn3/1 -> Vfn_pu/1  "Vfn_pu"
  IC1/1 -> Lag-lead network Transient gain reduction/1

== system myLibrary/SG_step/Exciter/Exciter ST4B ==
  note: Excitation
      | Control
      | Elements
  V_REF : Inport  SampleTime=Ts
  V_S : Inport  Port=2  SampleTime=Ts
  V_T : Inport  Port=3  SampleTime=Ts
  Ifd_pu : Inport  Port=4  SampleTime=Ts
  Fex : Subsystem  mask{K_C=K_C}
      mask prompts: K_C "Rectifier regulation factor, K_C (pu):"
  PI_M : Subsystem
  PI_R : Subsystem
  Product : Product  OutDataTypeStr=Inherit: Same as first input
  Product1 : Product
  Subsystem1 : Subsystem
      mask Display: disp('V_E=|K_P*V_T+j(K_I+K_P*X_L)*I_T|')
  Sum : Sum  Inputs=+-+  InputSameDT=on  SaturateOnIntegerOverflow=on  OutDataTypeStr=Inherit: Same as first input
  Transfer Fcn3 : TransferFcn  Denominator=[T_SG.exc.TA 1]
  V_T1 : InportShadow  Port=3  SampleTime=Ts
  Voltage transducer : spsFirstOrderFilterLib/First-Order Filter  FilterType=Lowpass  Tc=T_SG.exc.TR  Ts=sim_config.Ts  Initialize=on  Vac_Init=[0, 0, T_SG.fb]  Vdc_Init=initSG.Vref  PlotResponse=off  FreqRange="[0,  200,  1]"
  Efd_pu : Outport  VectorParamsAs1DForOutWhenUnconnected=off
  wires:
  V_REF/1 -> Sum/1
  V_T/1 -> Voltage transducer/1
  Sum/1 -> PI_R/1(u)
  Transfer Fcn3/1 -> Product/1  "V_A"
  Product/1 -> Efd_pu/1
  Fex/1(F_EX) -> Product1/1  "F_EX"
  V_T1/1 -> Subsystem1/1(V_T)
  Ifd_pu/1 -> Fex/2(Ifd)
  Subsystem1/1(y) -> Product1/2, Fex/1(V_E)  "V_E"
  Product1/1 -> Product/2  "V_B"
  V_S/1 -> Sum/3
  Voltage transducer/1 -> Sum/2  "Vc"
  PI_R/1(y) -> PI_M/1(u)  "V_R"
  PI_M/1(y) -> Transfer Fcn3/1  "V_M"

== system myLibrary/SG_step/Exciter/PSS 2A ==
  Vsi1 : Inport
  Vsi2 : Inport  Port=2
  DW{,1..5,7..8} (8 alike) : Scope
  Gain : Gain  Gain=ks3
  Gain1 : Gain  Gain=ks1
  LTI System1 : cstblocks/LTI System  sys=(tf([T8 1],1)/(tf([T9 1],1)^M))^N  IC=[]  PadeOrder=0
  Ramp-Tracking Filter : eeSmPSS2C/SM PSS2C/Ramp-Tracking Filter  Commented=on  T1=T_8  T2=T_9  M=M  N=N  Ts=Ts
  Sum : Sum  Inputs=|++
  Sum1 : Sum  Inputs=|+-
  Transfer Fcn : TransferFcn  Numerator="[Tw1  0]"  Denominator="[Tw1  1]"
  Transfer Fcn1 : TransferFcn  Numerator="[Tw2  0]"  Denominator=[Tw2 1]
  Transfer Fcn2 : TransferFcn  Numerator=[Tw3 0]  Denominator=[Tw3 1]
  Transfer Fcn3 : TransferFcn  Denominator=[T6 1]
  Transfer Fcn8 : TransferFcn  Numerator=[ks2]  Denominator="[T7  1]"
  t1,t2 : TransferFcn  Numerator=[T1 1]  Denominator=[T2 1]
  t3,t4 : TransferFcn  Numerator=[T3 1]  Denominator=[T4 1]
  Vst : Outport
  wires:
  Transfer Fcn3/1 -> DW8/1, Sum/1
  Transfer Fcn/1 -> Transfer Fcn1/1
  Vsi2/1 -> Transfer Fcn2/1
  Gain/1 -> Sum/2
  Transfer Fcn8/1 -> Sum1/2, Gain/1, DW1/1
  Transfer Fcn1/1 -> Transfer Fcn3/1
  Transfer Fcn2/1 -> Transfer Fcn8/1
  t3,t4/1 -> DW5/1, Vst/1
  Gain1/1 -> t1,t2/1, DW3/1
  t1,t2/1 -> t3,t4/1, DW4/1
  Sum/1 -> DW/1, LTI System1/1
  LTI System1/1 -> DW2/1, Sum1/1
  Vsi1/1 -> DW7/1, Transfer Fcn/1
  Sum1/1 -> Gain1/1

== system myLibrary/SG_step/Exciter/Terminal voltage magnitude ==
  Vq : Inport
  Vd : Inport  Port=2
  Add10 : Sum
  Product : Product
  Product1 : Product
  Square Root : Sqrt
  Vt : Outport
  wires:
  Product/1 -> Add10/1
  Vd/1 -> Product1/2, Product1/1
  Product1/1 -> Add10/2
  Add10/1 -> Square Root/1
  Vq/1 -> Product/1, Product/2
  Square Root/1 -> Vt/1  "V"

== system myLibrary/SG_step/Governor-Turbine/IEEEG1 ==
  speed_pu : Inport  SampleTime=Ts
  Pref : Inport  Port=2  SampleTime=Ts
  Add1 : Sum
  Constant : Constant  Value=pu_speed_reference
  Gain : Gain  Gain=K
  Gain10 : Gain  Gain=1/T_3
  Gain2 : Gain  Gain=K_2
  Gain3 : Gain  Gain=K_4
  Gain4 : Gain  Gain=K_6
  Gain5 : Gain  Gain=K_8
  Gain6 : Gain  Gain=K_1
  Gain7 : Gain  Gain=K_3
  Gain8 : Gain  Gain=K_5
  Gain9 : Gain  Gain=K_7
  Integrator : Integrator  InitialCondition=pu_torque0
  Lead-Lag : eeGeneralControl/Lead-Lag (Discrete or Continuous)  T1=T_2  T2=T_1  B=inf  A=-inf  init_option=Inherited from block input  x0=0  Ts=Ts
  Low-Pass Filter : eeGeneralControl/Low-Pass Filter (Discrete or Continuous)  K=1  T=T_4  B=inf  A=-inf  init_option=Inherited from block input  x0=0  Ts=Ts
  Low-Pass Filter1 : eeGeneralControl/Low-Pass Filter (Discrete or Continuous)  K=1  T=T_5  B=inf  A=-inf  init_option=Inherited from block input  x0=0  Ts=Ts
  Low-Pass Filter2 : eeGeneralControl/Low-Pass Filter (Discrete or Continuous)  K=1  T=T_6  B=inf  A=-inf  init_option=Inherited from block input  x0=0  Ts=Ts
  Low-Pass Filter3 : eeGeneralControl/Low-Pass Filter (Discrete or Continuous)  K=1  T=T_7  B=inf  A=-inf  init_option=Inherited from block input  x0=0  Ts=Ts
  Sum1 : Sum  Inputs=++-
  Sum2 : Sum  Inputs=|-+  OutDataTypeStr=Inherit: Same as first input
  Sum3 : Sum  Inputs=++|
  Sum4 : Sum  Inputs=++|
  Sum5 : Sum  Inputs=++|
  Sum6 : Sum  Inputs=|++
  Sum7 : Sum  Inputs=|++
  Sum8 : Sum  Inputs=|++
  Pm(HP) : Outport  VectorParamsAs1DForOutWhenUnconnected=off
  Pm(LP) : Outport  Port=2  VectorParamsAs1DForOutWhenUnconnected=off
  Pm : Outport  Port=3  VectorParamsAs1DForOutWhenUnconnected=off
  wires:
  Add1/1 -> Pm/1  "Pm"
  Gain10/1 -> Integrator/1
  Sum1/1 -> Gain10/1
  Constant/1 -> Sum2/2
  speed_pu/1 -> Sum2/1
  Sum5/1 -> Pm(LP)/1, Add1/2
  Sum8/1 -> Pm(HP)/1, Add1/1
  Sum7/1 -> Sum8/1
  Gain9/1 -> Sum8/2
  Sum6/1 -> Sum7/1
  Gain8/1 -> Sum7/2
  Gain5/1 -> Sum5/1
  Sum4/1 -> Sum5/2
  Sum3/1 -> Sum4/2
  Gain4/1 -> Sum4/1
  Gain2/1 -> Sum3/2
  Gain3/1 -> Sum3/1
  Gain7/1 -> Sum6/2
  Gain6/1 -> Sum6/1
  Low-Pass Filter3/1 -> Gain9/1, Gain5/1
  Low-Pass Filter1/1 -> Low-Pass Filter2/1, Gain3/1, Gain7/1
  Low-Pass Filter2/1 -> Low-Pass Filter3/1, Gain4/1, Gain8/1
  Low-Pass Filter/1 -> Gain2/1, Low-Pass Filter1/1, Gain6/1
  Pref/1 -> Sum1/1
  Integrator/1 -> Low-Pass Filter/1, Sum1/3
  Lead-Lag/1 -> Sum1/2
  Gain/1 -> Lead-Lag/1
  Sum2/1 -> Gain/1
